simulink model "quad_simulation_with_payload"  (R2021a)
settings: Solver=FixedStepAuto  StartTime=0.0  StopTime=sim_time  FixedStep=1/sim_freq  RelTol=1e-3
values from neighbouring files (symbols this model uses):
  hover_T_init = hover_init * max_total_T / 4    [initialize_quad_simulation.m]
libraries: simulink x2
settings Model: Creator=francois  LastModifiedBy=esl
settings SolverCC: AlgebraicLoopSolver=TrustRegion
settings DebuggingCC: ReadBeforeWriteMsg=DisableAll  WriteAfterWriteMsg=DisableAll  WriteAfterReadMsg=DisableAll  UniqueDataStoreMsg=error  StrictBusMsg=WarnOnBusTreatedAsVector  NonBusSignalsTreatedAsBus=warning  SFMachineParentedDataDiag=warning
settings ModelReferenceCC: UpdateModelReferenceTargets=IfOutOfDate  EnableParallelModelReferenceBuilds=on
settings SFSimCC: SFSimEcho=off

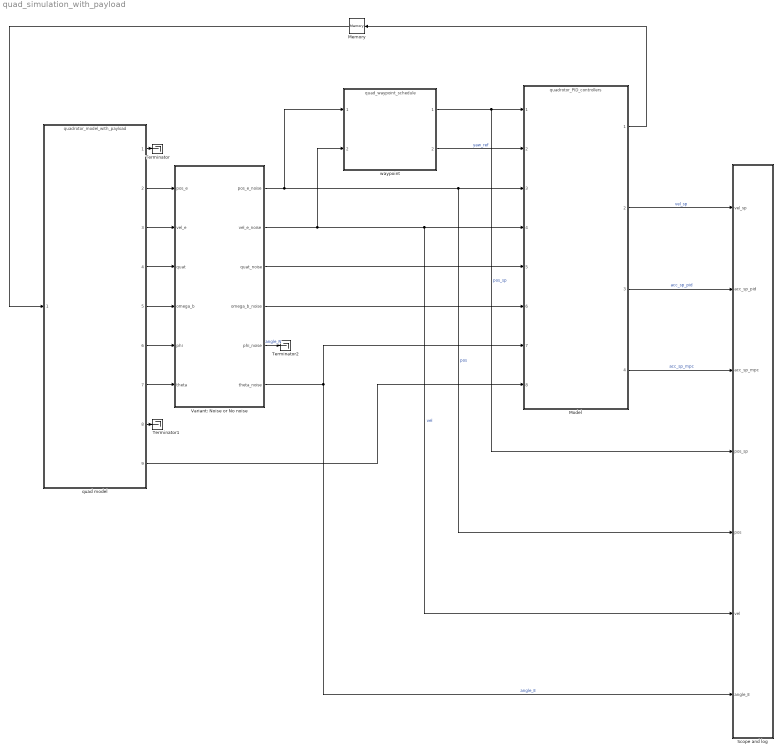
== system quad_simulation_with_payload ==
  Memory : Memory  InitialCondition=hover_T_init*ones(4,1)
  Model : ModelReference  ModelNameDialog=quadrotor_PID_controllers.slx  SimulationMode=Normal  ModelReferenceVersion=3.108
  Scope and log : Subsystem  TreatAsAtomicUnit=on
  Terminator : Terminator
  Terminator1 : Terminator
  Terminator2 : Terminator
  Variant: Noise or No noise : Subsystem  Variant=on
  quad model : ModelReference  ModelNameDialog=quadrotor_model_with_payload.slx  SimulationMode=Normal  ModelReferenceVersion=3.12
  waypoint : ModelReference  ModelNameDialog=quad_waypoint_schedule.slx  SimulationMode=Normal  ModelReferenceVersion=3.13
  wires:
  Variant: Noise or No noise/4(omega_b_noise) -> Model/6
  waypoint/2 -> Model/2  "yaw_ref"
  quad model/3 -> Variant: Noise or No noise/2(vel_e)
  Variant: Noise or No noise/2(vel_e_noise) -> waypoint/2, Scope and log/6(vel), Model/4  "vel"
  Variant: Noise or No noise/1(pos_e_noise) -> waypoint/1, Scope and log/5(pos), Model/3  "pos"
  quad model/5 -> Variant: Noise or No noise/4(omega_b)
  Variant: Noise or No noise/3(quat_noise) -> Model/5
  Memory/1 -> quad model/1
  quad model/1 -> Terminator/1
  Model/1 -> Memory/1
  waypoint/1 -> Scope and log/4(pos_sp), Model/1  "pos_sp"
  quad model/2 -> Variant: Noise or No noise/1(pos_e)
  quad model/4 -> Variant: Noise or No noise/3(quat)
  quad model/6 -> Variant: Noise or No noise/5(phi)
  Variant: Noise or No noise/6(theta_noise) -> Scope and log/7(angle_E), Model/7  "angle_E"
  quad model/7 -> Variant: Noise or No noise/6(theta)
  quad model/8 -> Terminator1/1
  Model/2 -> Scope and log/1(vel_sp)  "vel_sp"
  Model/3 -> Scope and log/2(acc_sp_pid)  "acc_sp_pid"
  Model/4 -> Scope and log/3(acc_sp_mpc)  "acc_sp_mpc"
  quad model/9 -> Model/8
  Variant: Noise or No noise/5(phi_noise) -> Terminator2/1  "angle_N"

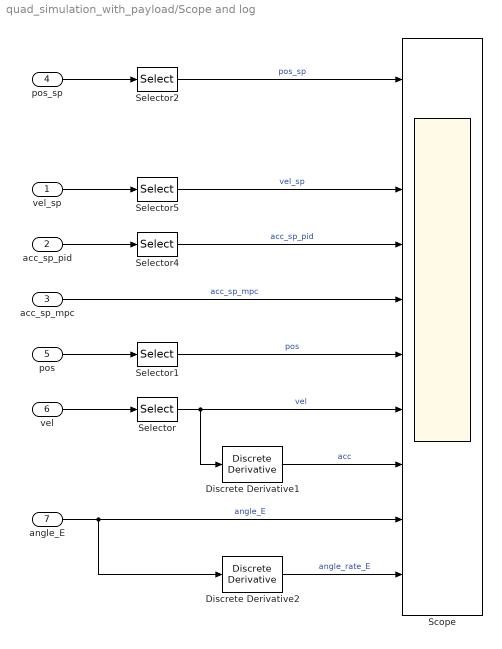
== system quad_simulation_with_payload/Scope and log ==
  vel_sp : Inport
  acc_sp_pid : Inport  Port=2
  acc_sp_mpc : Inport  Port=3
  pos_sp : Inport  Port=4
  pos : Inport  Port=5
  vel : Inport  Port=6
  angle_E : Inport  Port=7
  Discrete Derivative1 : simulink/Discrete/Discrete Derivative  gainval=1.0  ICPrevScaledInput=0.0  OutMin=[]  OutMax=[]  OutDataType=fixdt(1, 16)  OutScaling=2^-10  DoSatur=off
  Discrete Derivative2 : simulink/Discrete/Discrete Derivative  gainval=1.0  ICPrevScaledInput=0.0  OutMin=[]  OutMax=[]  OutDataType=fixdt(1, 16)  OutScaling=2^-10  DoSatur=off
  Scope : Scope  NumInputPorts=10
  Selector{,1..2,4..5} (5 alike) : Selector  InputPortWidth=3  IndexOptions=Index vector (dialog)  Indices=1  OutputSizes=1
  wires:
  Selector1/1 -> Scope/6  "pos"
  Selector/1 -> Scope/7, Discrete Derivative1/1  "vel"
  Selector4/1 -> Scope/4  "acc_sp_pid"
  angle_E/1 -> Discrete Derivative2/1, Scope/9  "angle_E"
  Selector5/1 -> Scope/3  "vel_sp"
  Selector2/1 -> Scope/1  "pos_sp"
  vel/1 -> Selector/1
  Discrete Derivative1/1 -> Scope/8  "acc"
  pos/1 -> Selector1/1
  acc_sp_pid/1 -> Selector4/1
  vel_sp/1 -> Selector5/1
  pos_sp/1 -> Selector2/1
  acc_sp_mpc/1 -> Scope/5  "acc_sp_mpc"
  Discrete Derivative2/1 -> Scope/10  "angle_rate_E"

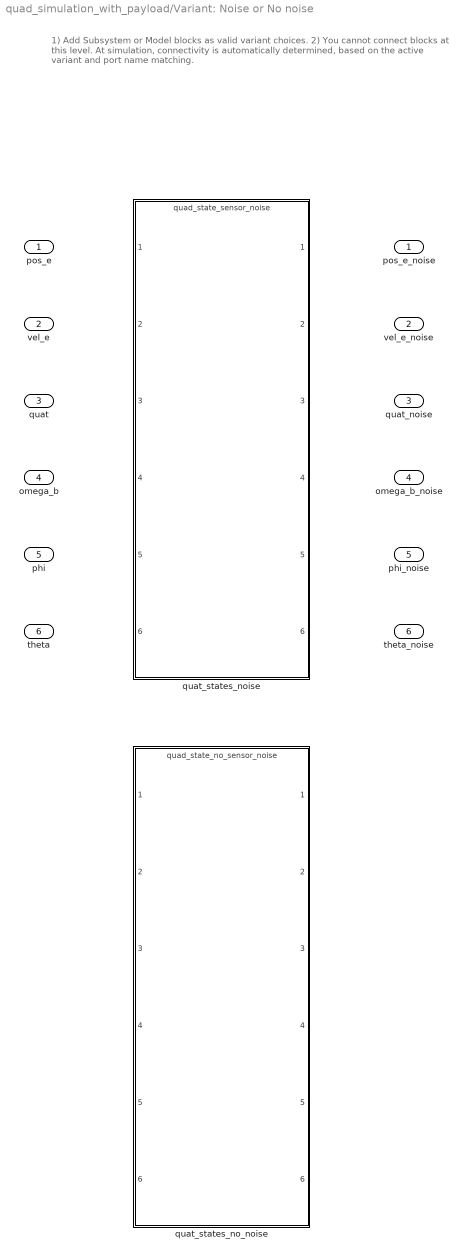
== system quad_simulation_with_payload/Variant: Noise or No noise ==
  note: 1) Add Subsystem or Model blocks as valid variant choices.
      | 2) You cannot connect blocks at this level. At simulation, connectivity is automatically
      | determined, based on the active variant and port name matching.
  pos_e : Inport  PortDimensions=3
  vel_e : Inport  Port=2  PortDimensions=3
  quat : Inport  Port=3  PortDimensions=4
  omega_b : Inport  Port=4  PortDimensions=3
  phi : Inport  Port=5  PortDimensions=1
  theta : Inport  Port=6  PortDimensions=1
  quat_states_no_noise : ModelReference  ModelNameDialog=quad_state_no_sensor_noise.slx  SimulationMode=Normal  VariantControl=no_noise_variant  ModelReferenceVersion=4.4
  quat_states_noise : ModelReference  ModelNameDialog=quad_state_sensor_noise.slx  SimulationMode=Normal  VariantControl=noise_variant  ModelReferenceVersion=3.2
  pos_e_noise : Outport  PortDimensions=3  VectorParamsAs1DForOutWhenUnconnected=off
  vel_e_noise : Outport  Port=2  PortDimensions=3  VectorParamsAs1DForOutWhenUnconnected=off
  quat_noise : Outport  Port=3  PortDimensions=4  VectorParamsAs1DForOutWhenUnconnected=off
  omega_b_noise : Outport  Port=4  PortDimensions=3  VectorParamsAs1DForOutWhenUnconnected=off
  phi_noise : Outport  Port=5  VectorParamsAs1DForOutWhenUnconnected=off
  theta_noise : Outport  Port=6  VectorParamsAs1DForOutWhenUnconnected=off
